simulink model "rt_test_c_tuning"  (R2019b)
settings: Solver=ode5  StartTime=0.0  StopTime=120  RelTol=1e-3
undefined symbols (not defined in the file): Standard_Devices, UDP_Protocol
libraries: fod x3, sldrtlib x2
settings Model: SimulationMode=external  ExtModeTrigDuration=250000  Creator=Aleksei  LastModifiedBy=Aleksei
settings DataIOCC: ReturnWorkspaceOutputs=off
settings DebuggingCC: ArithmeticOperatorsInVariantConditions=warning
settings SFSimCC: CustomCodeUndefinedFunction=UseInterfaceOnly
settings RTWCC: Description=Simulink Desktop Real-Time  SystemTargetFile=sldrt.tlc  TemplateMakefile=sldrt.tmf  RTWCompilerOptimization=on
settings CodeAppCC: MaxIdLength=95
settings SimulinkDesktopRealTimeCC: TargetPreCompLibLocation=C:\Program Files\MATLAB\R2019b\toolbox\sldrt\lib\win64  PreserveStateflowLocalDataDimensions=off

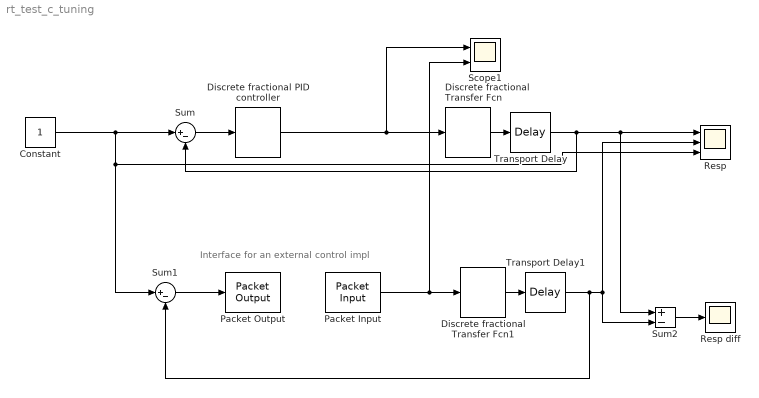
== system rt_test_c_tuning ==
  note: Interface for an external control impl
  Constant : Constant
  Discrete fractional PID controller : fod/Discrete fractional PID controller  Kp=0.017269125731976614  Ki=0.017405775915692517  lambda=0.8  Kd=0.033540278712465128  mu=0.4  freqRange=[0.001; 1000]  N=5  useRef=off  dscrMethod=Matched  wc=0  ts=0.01
      settings: SourceProductName=FOMCON Toolbox
  Discrete fractional Transfer Fcn : fod/Discrete fractional Transfer Fcn  zeroPoly=66.16  polePoly=12.72s^0.5+1  freqRange=[0.0001, 10000]  approxNum=5  useRef=off  dscrMethod=Matched  wc=0  ts=0.01
      settings: SourceProductName=FOMCON Toolbox
  Discrete fractional Transfer Fcn1 : fod/Discrete fractional Transfer Fcn  zeroPoly=66.16  polePoly=12.72s^0.5+1  freqRange=[0.0001, 10000]  approxNum=5  useRef=off  dscrMethod=Matched  wc=0  ts=0.01
      settings: SourceProductName=FOMCON Toolbox
  Packet Input : sldrtlib/Packet Input  SampleTime=0.01  MaxMissedTicks=10  ShowMissedTicks=off  YieldWhenWaiting=off  DrvName=Standard_Devices/UDP_Protocol  DrvAddress=5101  DrvOptions=[0 5111 49 50 55 46 48 46 48 46 49 0 0 0 0 0 0 0 0 0 0 0 0 0 0 0 0 0 0 0 0 0 0 0 0 0 0 0 0 0 0 0 0 0 0 0 0 0 0 0 0 0 0 0 0 0 0 0 0 0 0 0 0 0 0 0 0 0 0 0 0 0 0 0 0 0 0 0 0 0 0 0 0 0 0 0 0 0 0 0 0 0 0 0 0 0 0 0 0 0 0 0 0 0 0 0 0 0 0 0 0 0 0 0 0 0 0 0 0 0 0 0 0 0 0 0 0 0 0 0 0 0 0 0 0 0 0 0 0 0 0 0 0 0 0 0 0 0 0 0 0 0 0 0 0 0 0 0 0 0 0 0 0 0 0 0 0 0 0 0 0 0 0 0 0 0 0 0 0 0 0 0 0 0 0 0 0 0 0 0 0 0 0 0 0 0 0 0 0 0 0 0 0 0 0 0 0 0 0 0 0 0 0 0 0 0 0 0 0 0 0 0 0 0 0 0 0 0 0 0 0 0 0 0 0 0 0 0 0 0 0 0 0 0 0 0 0 0 0 0 0 0 0 0 0 0]  PacketSize=8  DataTypes='1*double'  ShowReady=off  ShowError=off  PacketID=1  ByteOrder=1  ShowTimestamp=off
      settings: AttributesFormatString=UDP Protocol [5101]  SourceProductName=Simulink Desktop Real-Time
  Packet Output : sldrtlib/Packet Output  SampleTime=0.01  MaxMissedTicks=10  ShowMissedTicks=off  YieldWhenWaiting=off  DrvName=Standard_Devices/UDP_Protocol  DrvAddress=5100  DrvOptions=[0 5110 49 50 55 46 48 46 48 46 49 0 0 0 0 0 0 0 0 0 0 0 0 0 0 0 0 0 0 0 0 0 0 0 0 0 0 0 0 0 0 0 0 0 0 0 0 0 0 0 0 0 0 0 0 0 0 0 0 0 0 0 0 0 0 0 0 0 0 0 0 0 0 0 0 0 0 0 0 0 0 0 0 0 0 0 0 0 0 0 0 0 0 0 0 0 0 0 0 0 0 0 0 0 0 0 0 0 0 0 0 0 0 0 0 0 0 0 0 0 0 0 0 0 0 0 0 0 0 0 0 0 0 0 0 0 0 0 0 0 0 0 0 0 0 0 0 0 0 0 0 0 0 0 0 0 0 0 0 0 0 0 0 0 0 0 0 0 0 0 0 0 0 0 0 0 0 0 0 0 0 0 0 0 0 0 0 0 0 0 0 0 0 0 0 0 0 0 0 0 0 0 0 0 0 0 0 0 0 0 0 0 0 0 0 0 0 0 0 0 0 0 0 0 0 0 0 0 0 0 0 0 0 0 0 0 0 0 0 0 0 0 0 0 0 0 0 0 0 0 0 0 0 0 0 0]  PacketSize=8  DataTypes='1*double'  ShowReady=off  ShowError=off  PacketID=1  ByteOrder=1  InitialValue=[]  FinalValue=[]
      settings: AttributesFormatString=UDP Protocol [5100]  SourceProductName=Simulink Desktop Real-Time
  Resp : Scope  NumInputPorts=3
  Resp diff : Scope
  Scope1 : Scope  NumInputPorts=2
  Sum : Sum  Inputs=|+-
  Sum1 : Sum  Inputs=|+-
  Sum2 : Sum  Inputs=+-
  Transport Delay : TransportDelay  DelayTime=1.93
  Transport Delay1 : TransportDelay  DelayTime=1.93
  wires:
  Transport Delay1/1 -> Sum1/2, Resp/2, Sum2/2
  Transport Delay/1 -> Sum/2, Sum2/1, Resp/1
  Constant/1 -> Resp/3, Sum1/1, Sum/1
  Sum1/1 -> Packet Output/1
  Packet Input/1 -> Discrete fractional Transfer Fcn1/1, Scope1/2
  Discrete fractional PID controller/1 -> Discrete fractional Transfer Fcn/1, Scope1/1
  Sum/1 -> Discrete fractional PID controller/1
  Sum2/1 -> Resp diff/1
  Discrete fractional Transfer Fcn/1 -> Transport Delay/1
  Discrete fractional Transfer Fcn1/1 -> Transport Delay1/1
